simulink library "yoshimuLibrary"  (R2018a)
settings: Solver=VariableStepAuto  StartTime=0.0  StopTime=10.0  RelTol=1e-3
undefined symbols (not defined in the file or in its folder): RE, RS
settings Model: Creator=yyas16  LastModifiedBy=yyas16

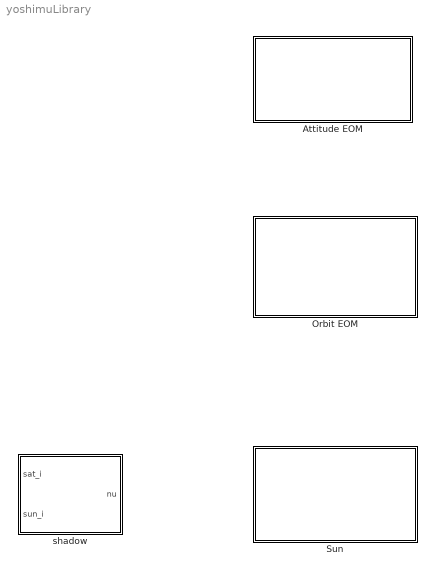
== system yoshimuLibrary ==
  Attitude EOM : Subsystem
  "Orbit EOM " : Subsystem
  Sun : Subsystem
      mask Display: image('sun.jpg');
  shadow : MATLAB Function  TreatAsAtomicUnit=on

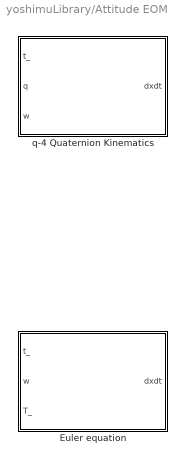
== system yoshimuLibrary/Attitude EOM ==
  Euler equation : MATLAB Function  TreatAsAtomicUnit=on
  q-4 Quaternion Kinematics : MATLAB Function  TreatAsAtomicUnit=on

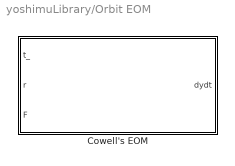
== system yoshimuLibrary/Orbit EOM  ==
  Cowell's EOM : MATLAB Function  TreatAsAtomicUnit=on

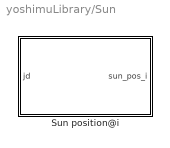
== system yoshimuLibrary/Sun ==
  Sun position@i : MATLAB Function  TreatAsAtomicUnit=on

== matlab function yoshimuLibrary/Attitude EOM/Euler equation ==
  data: dxdt output; t_ input; w input; T_ input; MOI parameter
function dxdt = eulerEOM(t_, w, T_, MOI)
% ----------------------------------------------------------------------
%   Equations of motion
%    20190214  y.yoshimura
%    Inputs: t_: time, s
%            x_: state variables
%   Outputs:
%   related function files:
%   note:
%   cf:
%   revisions;
%   
%   (c) 2019 yasuhiro yoshimura
%----------------------------------------------------------------------

%% state variables and inputs


%% equations of motion 
% do not rewrite the following script
dxdt = MOI^(-1) * (cross(-w, MOI*w) + T_);
end

== matlab function yoshimuLibrary/Orbit EOM /Cowell's EOM ==
  data: t_ input; dydt output; r input; F input; GE parameter
function dydt = cowellEOM(t_, r, F, GE)
% ----------------------------------------------------------------------
%   Equations of motion
%    20190214  y.yoshimura
%    Inputs: t_: time, s
%            x_: state variables
%   Outputs:
%   related function files:
%   note:
%   cf:
%   revisions;
%   
%   (c) 2019 yasuhiro yoshimura
%----------------------------------------------------------------------

%% state variables and inputs
r = r(:);
F = F(:);
% r = [x; y; z];
% v = [vx; vy; vz];

%% equations of motion 
% do not rewrite the following script
dydt = -GE ./ norm(r)^3 .* r + F;

end

== matlab function yoshimuLibrary/Attitude EOM/q-4 Quaternion Kinematics ==
  data: t_ input; dxdt output; q input; w input
function dxdt = q4Quaternion(t_, q, w)
% ----------------------------------------------------------------------
%   Equations of motion
%    20190214  y.yoshimura
%    Inputs: t_: time, s
%            q_: quaternion, q4 is scalar part
%            w: angular rate, rad/s
%   Outputs:
%   related function files:
%   note:
%   cf:
%   revisions;
%   
%   (c) 2019 yasuhiro yoshimura
%----------------------------------------------------------------------

%% state variables and inputs


%% equations of motion 
% do not rewrite the following script
dxdt = 0.5 .* qMult(4, 1, [w' 0], q')';
end

== matlab function yoshimuLibrary/Sun/Sun position@i ==
  data: jd input; sun_pos_i output; earthVSOP parameter
function sun_pos_i = sunPos(jd, earthVSOP)
% ----------------------------------------------------------------------
%    Sun position at inertial frame
%    20190227  y.yoshimura
%    Inputs: t, s,
%            jd, Julian day, day
%   Outputs: sun_pos_i: Sun position at inertial frame, km
%   related function files:
%   note:
%   cf:
%   revisions;
%   
%   (c) 2019 yasuhiro yoshimura
%----------------------------------------------------------------------

[l_sun, b_sun, dis_sun] = sun(jd, earthVSOP);
sun_pos_i = lonLat2pos(l_sun, b_sun, AU2km(dis_sun));

== matlab function yoshimuLibrary/shadow ==
  data: sat_i input; nu output; sun_i input; RS parameter; RE parameter
function nu = shadowS(sat_i, sun_i, RS, RE)
% ----------------------------------------------------------------------
%   calculate shadow function
%    20190220  y.yoshimura
%    Inputs: sat_i, satellite position@inertial frame, nx3
%            sun_i, sun position@inertial frame, nx3
%   Outputs: nu, shadow coefficient, nx1 vector
%            nu == 1 sunlit
%            nu == 0 eclipse
%            0< nu <1: partial eclipse
%   related function files:
%   note:
%   cf: Satellite Orbits, Montenbruck, Gill, p.81
%   revisions;
%   function nu = shadow(sat_i, sun_i)
%   (c) 2019 yasuhiro yoshimura
%----------------------------------------------------------------------

nu = shadow(sat_i', sun_i, RE, RS); % calc shadow
